simulink model "the_last_domaci2_m2012"  (R2012a)
settings: Solver=ode45  StartTime=0.0  StopTime=10  RelTol=1e-3
values from neighbouring files (symbols this model uses):
  A = [1 a 0]    [main.m]
  Am = [1 alpha1 alpha0]    [main.m]
  B = [b]    [main.m]
  Bm = [alpha0]    [main.m]
  R = [1 r0]    [main.m]
  S = [p1 p0]    [main.m]
  T = [t1 t0]    [main.m]
  Ts = 0.01    [main.m]
settings Model: CovModelRefEnable=off  Creator=Vukan  LastModifiedBy=Vukan
settings DataIOCC: SaveFormat=StructureWithTime  ReturnWorkspaceOutputs=off
settings OptimizationCC: LifeSpan=inf  SimCompilerOptimization=Off
settings DebuggingCC: FcnCallInpInsideContextMsg=Enable All  SFUnexpectedBacktrackingDiag=warning  SFNoUnconditionalDefaultTransitionDiag=warning
settings HardwareCC: ProdWordSize=32  ProdHWDeviceType=Specified
settings SFSimCC: SimUseLocalCustomCode=off
settings RTWCC: RTWUseLocalCustomCode=off  RTWCompilerOptimization=Off
settings GRTTargetCC: CodeReplacementLibrary=C89/C90 (ANSI)  GeneratePreprocessorConditionals=Disable all  CPPClassGenCompliant=off

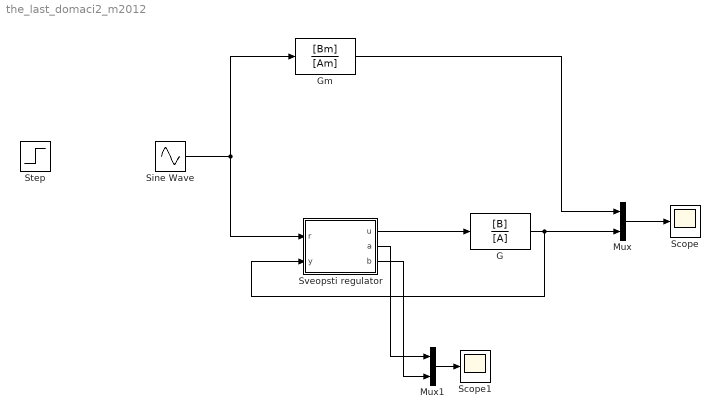
== system the_last_domaci2_m2012 ==
  G : TransferFcn  Numerator=[B]  Denominator=[A]
  Gm : TransferFcn  Numerator=[Bm]  Denominator=[Am]
  Mux : Mux  Inputs=2
  Mux1 : Mux  Inputs=2
  Scope : Scope
      settings: TimeRange=auto  MaxDataPoints=5000  SaveToWorkspace=off  SaveName=ScopeData  YMin=-0.12485  YMax=1.12361  SampleTime=-1
  Scope1 : Scope
      settings: TimeRange=auto  MaxDataPoints=5000  SaveToWorkspace=off  YMin=-2623552812563563900000000000000000000000000000000000000000000000000000000000000000000000000000000000000000000000000000000000000000000000000000000000000000000000000000000000000000000000000000000000000000000000000000000000000000000000000000000000000000000000000000000000000000000000000000000000.00000  YMax=23611975313072081000000000000000000000000000000000000000000000000000000000000000000000000000000000000000000000000000000000000000000000000000000000000000000000000000000000000000000000000000000000000000000000000000000000000000000000000000000000000000000000000000000000000000000000000000000000000.00000  SampleTime=-1
  Sine Wave : Sin  Frequency=2*pi  SampleTime=0
  Step : Step  SampleTime=0
  Sveopsti regulator : MATLAB Function  TreatAsAtomicUnit=on
      settings: PermitHierarchicalResolution=ParametersOnly
  wires:
  Sveopsti regulator/1(u) -> G/1
  G/1 -> Sveopsti regulator/2(y), Mux/2
  Sine Wave/1 -> Sveopsti regulator/1(r), Gm/1
  Mux/1 -> Scope/1
  Gm/1 -> Mux/1
  Mux1/1 -> Scope1/1
  Sveopsti regulator/3(b) -> Mux1/2
  Sveopsti regulator/2(a) -> Mux1/1

== matlab function the_last_domaci2_m2012/Sveopsti regulator ==
  settings: updateMethod=DISCRETE  sampleTime=Ts
  data: r input; u output; y input; R parameter; S parameter; T parameter; Ts parameter; a output; b output
function [u, a, b] = fcn(r, y, R, S, T, Ts)

lambda = 1;

persistent P;
if isempty(P)
    P = 10000*eye(2);
end

persistent yp_staro;
if isempty(yp_staro)
    yp_staro = 0;
end
persistent yf1_staro;
if isempty(yf1_staro)
    yf1_staro = 0;
end

% Filtering
q = 1/Ts;
yq = y * q*q;

ypp = yq + yf1_staro*(-q*q) + yp_staro * (-2*q); 
yp_staro = yp_staro + Ts*ypp;
yf1_staro = yf1_staro + Ts*yp_staro;


persistent rp_staro;
if isempty(rp_staro)
    rp_staro = 0;
end
persistent rf1_staro;
if isempty(rf1_staro)
    rf1_staro = 0;
end

persistent theta;
if isempty(theta)
    theta = [0 0]';
end

% Filtering
q = 1/Ts;
rq = r * q*q;
rpp = rq + rf1_staro*(-q*q) + rp_staro * (-2*q); 
rp_staro = rp_staro + Ts*rpp;
rf1_staro = rf1_staro + Ts*rp_staro;

z = ypp;
X = [-yp_staro rf1_staro]';

P = (1/lambda) * (P -   (P*X*X'*P) / (lambda + X'*P*X));
theta = theta + P*X*(yf1_staro - X'*theta);


ksi = 1;
w0 = 1;

alpha0 = w0*w0;
alpha1 = 2*ksi*w0;
alpha2 = 3; %STA OVDE

a = theta(1);
b = theta(2);

% % A = [1 a 0];
% % B = [b]; %#ok<*NBRAK>
% % 
% % Am = [1 alpha1 alpha0];
% % Bm = [alpha0];
% 
% r0 = (alpha1 + alpha2) - a;
% R = [1 r0];
% 
% p0 = alpha0*alpha2 / b;
% p1 = (alpha0 + alpha1*alpha2-a*r0)/b;
% S = [p1 p0];
% 
% t1 = alpha0/b;
% t0 = alpha2*alpha0/b;
% T = [t1 t0];
% 
% 
% % Feedback
% persistent yf;
% if isempty(yf)
%     yf = 0;
% end
% 
% yf_staro = yf;
% 
% p = exp(-R(2)*Ts);
% yf = p * yf_staro + (1-p)*y;
% ufb = (1/R(2)) * ((S(1)/Ts) * (yf - yf_staro) + S(2) * yf);
% 
% % Feedforward
% persistent rf;
% if isempty(rf)
%     rf = 0;
% end
% rf_staro = rf;
% 
% rf = p * rf_staro + (1-p)*r;
% uff = (1/R(2)) * ((T(1)/Ts) * (rf - rf_staro) + T(2) * rf);
% 
% u = uff - ufb;
u = 1;
